simulink model "moteur1109"  (R2023a)
settings: Solver=VariableStepAuto  StartTime=0.0  StopTime=0.5  FixedStep=0.0000001  RelTol=1e-9
values from neighbouring files (symbols this model uses):
  J = 83e-6    (= 8.3e-05)    [donnees_moteur.m]
  kphi = 0.127    [donnees_moteur.m]
  L = 2.2e-3    (= 0.0022)    [donnees_moteur.m]
  R = 1.52    [donnees_moteur.m]
settings Model: Creator=magic  LastModifiedBy=magic

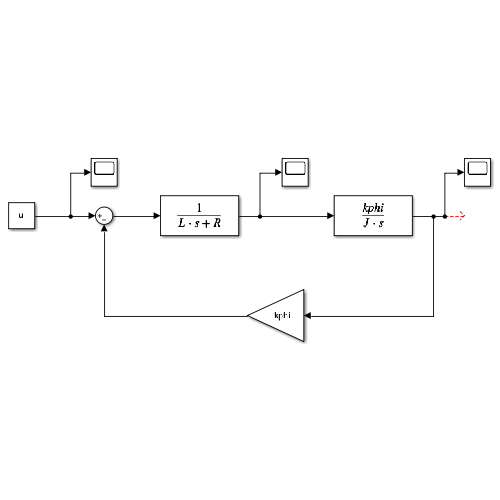
[thumbnail: Simulink's stored preview of the top-level diagram]
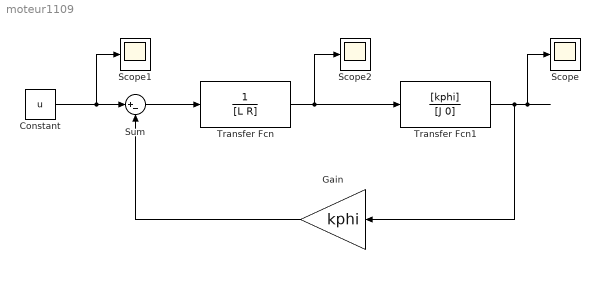
== system moteur1109 ==
  Constant : Constant  Value=u
  Gain : Gain  Gain=kphi
  Scope : Scope
  Scope1 : Scope
  Scope2 : Scope
  Sum : Sum  Inputs=|+-
  Transfer Fcn : TransferFcn  Denominator=[L R]
  Transfer Fcn1 : TransferFcn  Numerator=[kphi]  Denominator=[J 0]
  wires:
  Sum/1 -> Transfer Fcn/1
  Transfer Fcn/1 -> Scope2/1, Transfer Fcn1/1
  Transfer Fcn1/1 -> Scope/1, Gain/1
  Gain/1 -> Sum/2
  Constant/1 -> Scope1/1, Sum/1
